simulink model "VarDelayTesting"  (R2019b)
settings: Solver=FixedStepAuto  StartTime=0.0  StopTime=stop_time  FixedStep=Ts  RelTol=1e-3
InitFcn:
  | VarDelayInit
StopFcn:
  | VarDelayStop
values from neighbouring files (symbols this model uses):
  Ts = Ts*0.25    (= 5.20833333333e-06)    [VarDelayInit.m]
libraries: FPGA_Open_Speech_Tools x1
settings Model: Creator=Bailey  LastModifiedBy=Balad

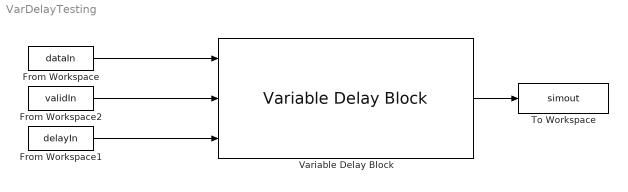
== system VarDelayTesting ==
  From Workspace : FromWorkspace  VariableName=dataIn  SampleTime=Ts
  From Workspace1 : FromWorkspace  VariableName=delayIn  SampleTime=Ts
  From Workspace2 : FromWorkspace  VariableName=validIn  SampleTime=Ts
  To Workspace : ToWorkspace  VariableName=simout  SaveFormat=Timeseries  SampleTime=-1
  Variable Delay Block : FPGA_Open_Speech_Tools/Variable Delay Block  maxDelay=8
  wires:
  From Workspace/1 -> Variable Delay Block/1
  From Workspace1/1 -> Variable Delay Block/3
  Variable Delay Block/1 -> To Workspace/1
  From Workspace2/1 -> Variable Delay Block/2
